simulink model "SRM_Project"  (R2025b)
settings: Solver=ode4  StartTime=0.0  StopTime=0.2  FixedStep=1e-5  RelTol=1e-3
InitFcn:
  | SRM_params
values from neighbouring files (symbols this model uses):
  B = 0.001    [SRM_params_template.m]
  delta_i = 0.1    [SRM_params_template.m]
  dLdth_vec = gradient(L_vec, theta_vec)    [SRM_params_template.m]
  Imax = 15    [SRM_params_template.m]
  J = 0.002    [SRM_params_template.m]
  Ki_w = 10    [SRM_params_template.m]
  Kp_w = 0.5    [SRM_params_template.m]
  L_vec = zeros(size(theta_vec))    [SRM_params_template.m]
  phase_offset = 2*pi/(Nph*Nr)    (= 0.523598775598)    [SRM_params_template.m]
  Rs = 1.0    (= 1)    [SRM_params_template.m]
  T_max = 5    [SRM_params_template.m]
  theta_off = deg2rad(38)    [SRM_params_template.m]
  theta_on = 0    [SRM_params_template.m]
  theta_ov = deg2rad(10)    [SRM_params_template.m]
  theta_vec = linspace(0, pi/2, 1000)    [SRM_params_template.m]
  TL = 1.5    [SRM_params_template.m]    (also in SRM_plots.m = out.TorqueData.signals(1).values(:, 2))
  tsf_type = 3    [SRM_params_template.m]
  Vdc = 300    [SRM_params_template.m]
libraries: slpidlib x1
settings Model: Creator=Dell  LastModifiedBy=Dell

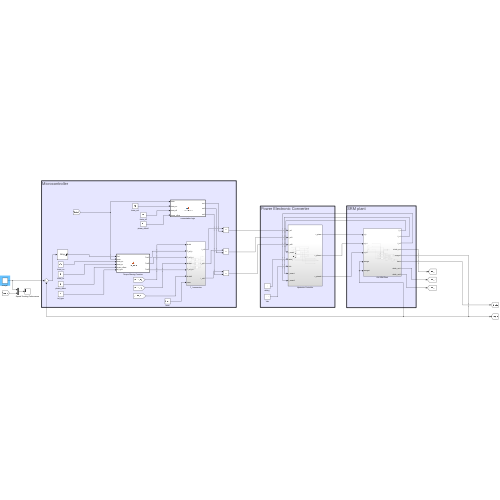
[thumbnail: Simulink's stored preview of the top-level diagram]
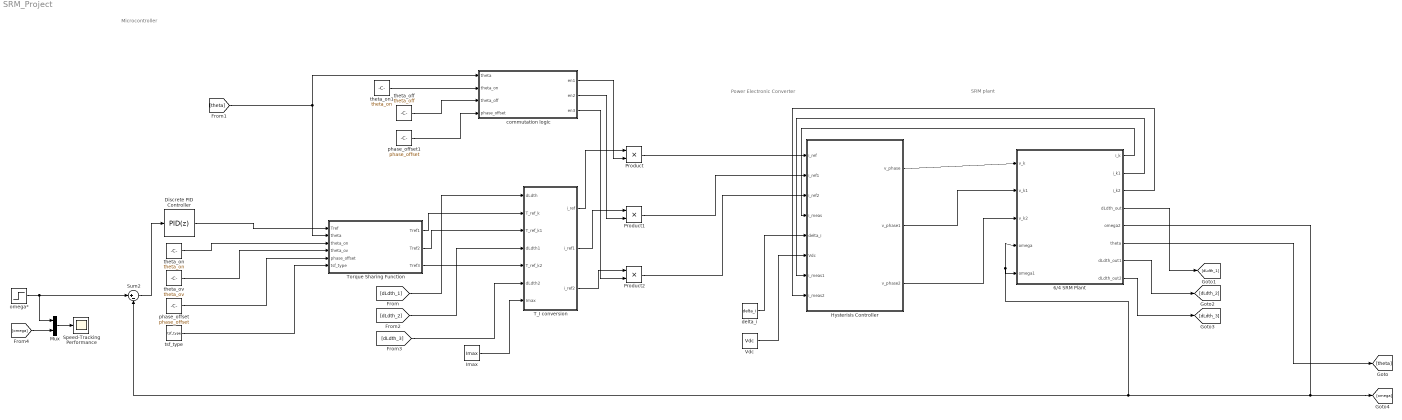
== system SRM_Project ==
  note: Power Electronic Converter
  note: Microcontroller
  note: SRM plant
  6/4 SRM Plant : Subsystem
  Discrete PID Controller : slpidlib/PID Controller  Controller=PID  Form=Parallel  TimeDomain=Discrete-time  UseExternalTs=off  SampleTime=-1  IntegratorMethod=Forward Euler  FilterMethod=Forward Euler  ControllerParametersSource=internal  P=Kp_w  I=Ki_w  UseKiTs=off  D=0  UseExternalDerivativeSource=off  N=100  UseFilter=on  TunerSelectOption=Transfer Function Based (PID Tuner App)  InitialConditionSource=internal  InitialConditionForIntegrator=0  InitialConditionForFilter=0  DifferentiatorICPrevScaledInput=0  ExternalReset=none  TrackingMode=off  Kt=1  LimitOutput=on  SatLimitsSource=internal  UpperSaturationLimit=T_max  LowerSaturationLimit=0  LinearizeAsGain=off  AntiWindupMode=none  Kb=1  LimitIntegrator=off  UpperIntegratorSaturationLimit=inf  LowerIntegratorSaturationLimit=-inf  POutMin=[]  POutMax=[]  IOutMin=[]  IOutMax=[]  DOutMin=[]  DOutMax=[]  NOutMin=[]  NOutMax=[]  SumOutMin=[]  SumOutMax=[]  SaturationOutMin=[]  SaturationOutMax=[]  PParamMin=[]  PParamMax=[]  IParamMin=[]  IParamMax=[]  DParamMin=[]  DParamMax=[]  NParamMin=[]  NParamMax=[]  KbParamMin=[]  KbParamMax=[]  KtParamMin=[]  KtParamMax=[]  KbOutMin=[]  KbOutMax=[]  KtOutMin=[]  KtOutMax=[]  IntegratorOutMin=[]  IntegratorOutMax=[]  FilterOutMin=[]  FilterOutMax=[]  SumI1OutMin=[]  SumI1OutMax=[]  SumI2OutMin=[]  SumI2OutMax=[]  SumI3OutMin=[]  SumI3OutMax=[]  SumI4OutMin=[]  SumI4OutMax=[]  SumDOutMin=[]  SumDOutMax=[]  DifferentiatorOutMin=[]  DifferentiatorOutMax=[]  FilterDiffOutCoefMin=[]  FilterDiffOutCoefMax=[]  ReciprocalOutMin=[]  ReciprocalOutMax=[]  SumDenOutMin=[]  SumDenOutMax=[]  SumNumOutMin=[]  SumNumOutMax=[]  DivideOutMin=[]  DivideOutMax=[]  UdiffTsProdOutMin=[]  UdiffTsProdOutMax=[]  NTsProdOutMin=[]  NTsProdOutMax=[]  UintegralTsProdOutMin=[]  UintegralTsProdOutMax=[]  UngainTsProdOutMin=[]  UngainTsProdOutMax=[]  ClampingZeroOutDataTypeStr=Inherit: Inherit via back propagation  ClampingZeroOutMin=[]  ClampingZeroOutMax=[]  FilterDenConstantOutDataTypeStr=Inherit: Inherit via back propagation  FilterDenConstantOutMin=[]  FilterDenConstantOutMax=[]  PCopyOutDataTypeStr=Inherit: Inherit via back propagation  PCopyOutMin=[]  PCopyOutMax=[]  NCopyOutDataTypeStr=Inherit: Inherit via back propagation  NCopyOutMin=[]  NCopyOutMax=[]  IntegratorContinuousStateAttributes=''  IntegratorStateMustResolveToSignalObject=off  IntegratorRTWStateStorageClass=Auto  FilterContinuousStateAttributes=''  FilterStateMustResolveToSignalObject=off  FilterRTWStateStorageClass=Auto  ParallelPVariant=InternalParameters  IdealPVariant=Disabled  IVariant=InternalParameters  DVariant=InternalParameters  IntegratorVariant=Discrete  SatVariant=Enabled  AWVariant=Passthrough  PCopyVariant=Disabled  TRVariant=Disabled  FdbkBlocksVariant=Forward  IdealPFdbkVariant=Disabled  SatFdbkVariant=Disabled  DerivativeFilterVariant=ForwardEulerFilter  NVariant=InternalParameters  NCopyVariant=Disabled  FilterICVariant=InternalICsFilter  IntegratorICVariant=InternalICs  ExternalResetVariant=Disabled  TRSumVariant=Passthrough  SumFdbkVariant=Disabled  SumVariant=Sum_PID  TsampFilterVariant=InternalTs  TsampNgainVariant=Passthrough  TsampIntegralVariant=Disabled_SignalSpec  ExternalSaturationOutDataTypeStr=Inherit: Same as second input  DerivativeSourceVariant=ErrorSignal  PreIntVariant=InternalPreInt
      settings: LibrarySourceBlock=simulink/Discrete/Discrete PID Controller
  Hysterisis Controller : Subsystem
  Imax : Constant  Value=Imax
  Mux : Mux  Inputs=2
  Product : Product
  Product1 : Product
  Product2 : Product
  Speed-Tracking Performance : Scope
      settings: Title=Speed Tracking Performance  ActiveDisplayYMinimum=-84.626335167126086  ActiveDisplayYMaximum=313.00000660773765  YLabel=Omega  DataLoggingVariableName=SpeedData
  Sum2 : Sum  Inputs=|+-
  T_I conversion : Subsystem
  Torque Sharing Function : MATLAB Function  TreatAsAtomicUnit=on
  Vdc : Constant  Value=Vdc
  commutation logic : MATLAB Function  TreatAsAtomicUnit=on
  delta_i : Constant  Value=delta_i
  omega* : Step  Time=0  After=100  SampleTime=0
  phase_offset : Constant  Value=phase_offset
  phase_offset1 : Constant  Value=phase_offset
  theta_off : Constant  Value=theta_off
  theta_on : Constant  Value=theta_on
  theta_on1 : Constant  Value=theta_on
  theta_ov : Constant  Value=theta_ov
  tsf_type : Constant  Value=tsf_type
  wires:
  omega*/1 -> Mux/1, Sum2/1
  Sum2/1 -> Discrete PID Controller/1
  Discrete PID Controller/1 -> Torque Sharing Function/1(Tref)
  commutation logic/1(en1) -> Product/2
  commutation logic/2(en2) -> Product1/2
  commutation logic/3(en3) -> Product2/2
  [theta] -> Torque Sharing Function/2(theta), commutation logic/1(theta)
  theta_on/1 -> Torque Sharing Function/3(theta_on)
  theta_ov/1 -> Torque Sharing Function/4(theta_ov)
  theta_on1/1 -> commutation logic/2(theta_on)
  phase_offset/1 -> Torque Sharing Function/5(phase_offset)
  phase_offset1/1 -> commutation logic/4(phase_offset)
  tsf_type/1 -> Torque Sharing Function/6(tsf_type)
  theta_off/1 -> commutation logic/3(theta_off)
  [omega] -> Mux/2
  Mux/1 -> Speed-Tracking Performance/1
  Product/1 -> Hysterisis Controller/1(i_ref)
  Product1/1 -> Hysterisis Controller/2(i_ref1)
  Product2/1 -> Hysterisis Controller/3(i_ref2)
  delta_i/1 -> Hysterisis Controller/5(delta_i)
  Vdc/1 -> Hysterisis Controller/6(Vdc)
  6/4 SRM Plant/5(omega2) -> [omega], 6/4 SRM Plant/4(omega), 6/4 SRM Plant/5(omega1), Sum2/2
  Hysterisis Controller/1(v_phase) -> 6/4 SRM Plant/1(v_k)
  Hysterisis Controller/2(v_phase1) -> 6/4 SRM Plant/2(v_k1)
  Hysterisis Controller/3(v_phase2) -> 6/4 SRM Plant/3(v_k2)
  6/4 SRM Plant/1(i_k) -> Hysterisis Controller/4(i_meas)
  6/4 SRM Plant/2(i_k1) -> Hysterisis Controller/7(i_meas1)
  6/4 SRM Plant/3(i_k2) -> Hysterisis Controller/8(i_meas2)
  6/4 SRM Plant/4(dLdth_out) -> [dLdth_1]
  6/4 SRM Plant/6(theta) -> [theta]
  6/4 SRM Plant/7(dLdth_out1) -> [dLdth_2]
  6/4 SRM Plant/8(dLdth_out2) -> [dLdth_3]
  [dLdth_1] -> T_I conversion/1(dLdth)
  Torque Sharing Function/1(Tref1) -> T_I conversion/2(T_ref_k)
  Torque Sharing Function/2(Tref2) -> T_I conversion/3(T_ref_k1)
  [dLdth_2] -> T_I conversion/4(dLdth1)
  Torque Sharing Function/3(Tref3) -> T_I conversion/5(T_ref_k2)
  [dLdth_3] -> T_I conversion/6(dLdth2)
  Imax/1 -> T_I conversion/7(Imax)
  T_I conversion/1(i_ref) -> Product/1
  T_I conversion/2(i_ref1) -> Product1/1
  T_I conversion/3(i_ref2) -> Product2/1

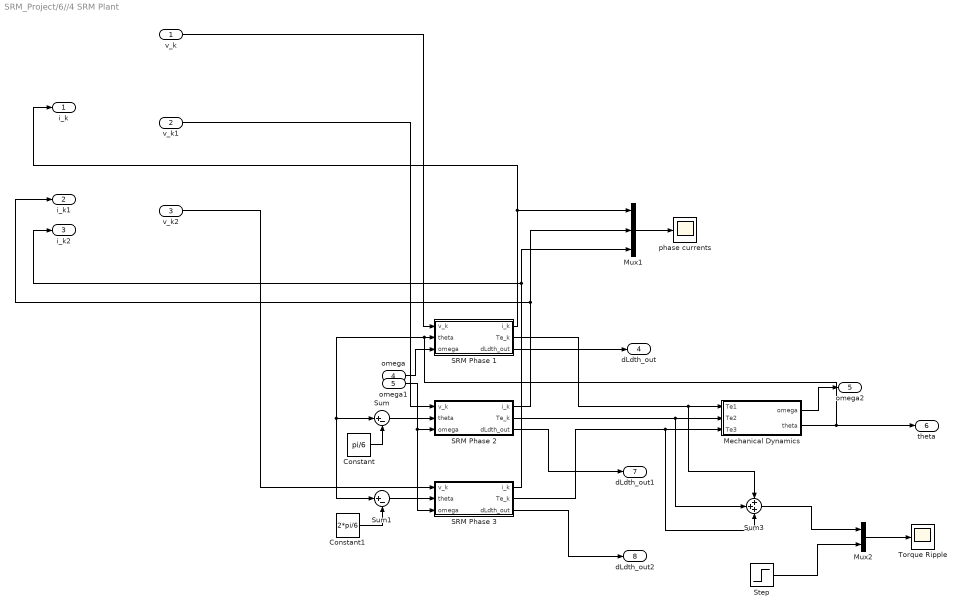
== system SRM_Project/6//4 SRM Plant ==
  v_k : Inport
  v_k1 : Inport  Port=2
  v_k2 : Inport  Port=3
  omega : Inport  Port=4
  omega1 : Inport  Port=5
  Constant : Constant  Value=pi/6
  Constant1 : Constant  Value=2*pi/6
  Mechanical Dynamics : Subsystem
  Mux1 : Mux  Inputs=3
  Mux2 : Mux  Inputs=2
  SRM Phase 1 : Subsystem
  SRM Phase 2 : Subsystem
  SRM Phase 3 : Subsystem
  Step : Step  Time=0.1  After=TL  SampleTime=0
  Sum : Sum  Inputs=|+-
  Sum1 : Sum  Inputs=|+-
  Sum3 : Sum  Inputs=+++
  Torque Ripple : Scope
      settings: ActiveDisplayYMinimum=-0.28454912524967474  ActiveDisplayYMaximum=2.8390389361123889  DataLoggingVariableName=TorqueData
  phase currents : Scope
      settings: ActiveDisplayYMinimum=-0.63560077718964481  ActiveDisplayYMaximum=5.7204069947068081  DataLoggingVariableName=CurrentData
  i_k : Outport
  i_k1 : Outport  Port=2
  i_k2 : Outport  Port=3
  dLdth_out : Outport  Port=4
  omega2 : Outport  Port=5
  theta : Outport  Port=6
  dLdth_out1 : Outport  Port=7
  dLdth_out2 : Outport  Port=8
  wires:
  Mechanical Dynamics/2(theta) -> theta/1, Sum/1, Sum1/1, SRM Phase 1/2(theta)
  Mux1/1 -> phase currents/1
  Sum1/1 -> SRM Phase 3/2(theta)
  SRM Phase 1/2(Te_k) -> Sum3/1, Mechanical Dynamics/1(Te1)
  v_k2/1 -> SRM Phase 3/1(v_k)
  SRM Phase 2/2(Te_k) -> Sum3/2, Mechanical Dynamics/2(Te2)
  Mechanical Dynamics/1(omega) -> omega2/1
  Sum/1 -> SRM Phase 2/2(theta)
  Constant1/1 -> Sum1/2
  Sum3/1 -> Mux2/1
  omega1/1 -> SRM Phase 3/3(omega), SRM Phase 2/3(omega)
  SRM Phase 3/1(i_k) -> i_k2/1, Mux1/3
  Constant/1 -> Sum/2
  SRM Phase 3/2(Te_k) -> Sum3/3, Mechanical Dynamics/3(Te3)
  Mux2/1 -> Torque Ripple/1
  SRM Phase 2/1(i_k) -> i_k1/1, Mux1/2
  SRM Phase 3/3(dLdth_out) -> dLdth_out2/1
  v_k1/1 -> SRM Phase 2/1(v_k)
  Step/1 -> Mux2/2
  SRM Phase 1/1(i_k) -> i_k/1, Mux1/1
  SRM Phase 1/3(dLdth_out) -> dLdth_out/1
  SRM Phase 2/3(dLdth_out) -> dLdth_out1/1
  omega/1 -> SRM Phase 1/3(omega)
  v_k/1 -> SRM Phase 1/1(v_k)

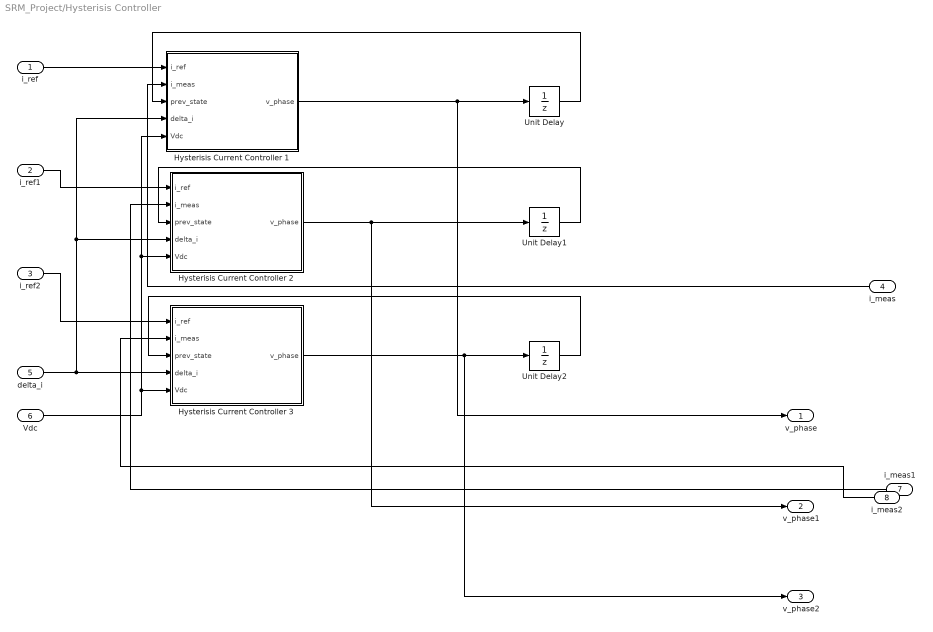
== system SRM_Project/Hysterisis Controller ==
  i_ref : Inport
  i_ref1 : Inport  Port=2
  i_ref2 : Inport  Port=3
  i_meas : Inport  Port=4
  delta_i : Inport  Port=5
  Vdc : Inport  Port=6
  i_meas1 : Inport  Port=7
  i_meas2 : Inport  Port=8
  Hysterisis Current Controller 1 : MATLAB Function  TreatAsAtomicUnit=on
  Hysterisis Current Controller 2 : MATLAB Function  TreatAsAtomicUnit=on
  Hysterisis Current Controller 3 : MATLAB Function  TreatAsAtomicUnit=on
  Unit Delay : UnitDelay  SampleTime=-1  HasFrameUpgradeWarning=on
  Unit Delay1 : UnitDelay  SampleTime=-1  HasFrameUpgradeWarning=on
  Unit Delay2 : UnitDelay  SampleTime=-1  HasFrameUpgradeWarning=on
  v_phase : Outport
  v_phase1 : Outport  Port=2
  v_phase2 : Outport  Port=3
  wires:
  Vdc/1 -> Hysterisis Current Controller 1/5(Vdc), Hysterisis Current Controller 2/5(Vdc), Hysterisis Current Controller 3/5(Vdc)
  Unit Delay1/1 -> Hysterisis Current Controller 2/3(prev_state)
  Hysterisis Current Controller 2/1(v_phase) -> v_phase1/1, Unit Delay1/1
  delta_i/1 -> Hysterisis Current Controller 3/4(delta_i), Hysterisis Current Controller 1/4(delta_i), Hysterisis Current Controller 2/4(delta_i)
  Hysterisis Current Controller 1/1(v_phase) -> v_phase/1, Unit Delay/1
  Unit Delay/1 -> Hysterisis Current Controller 1/3(prev_state)
  Hysterisis Current Controller 3/1(v_phase) -> v_phase2/1, Unit Delay2/1
  i_meas1/1 -> Hysterisis Current Controller 2/2(i_meas)
  i_ref1/1 -> Hysterisis Current Controller 2/1(i_ref)
  Unit Delay2/1 -> Hysterisis Current Controller 3/3(prev_state)
  i_ref/1 -> Hysterisis Current Controller 1/1(i_ref)
  i_ref2/1 -> Hysterisis Current Controller 3/1(i_ref)
  i_meas2/1 -> Hysterisis Current Controller 3/2(i_meas)
  i_meas/1 -> Hysterisis Current Controller 1/2(i_meas)

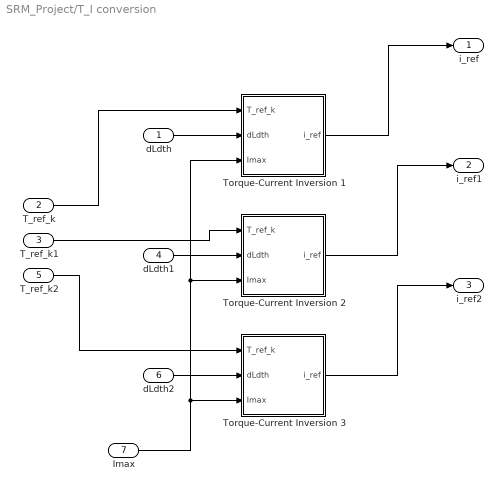
== system SRM_Project/T_I conversion ==
  dLdth : Inport
  T_ref_k : Inport  Port=2
  T_ref_k1 : Inport  Port=3
  dLdth1 : Inport  Port=4
  T_ref_k2 : Inport  Port=5
  dLdth2 : Inport  Port=6
  Imax : Inport  Port=7
  Torque-Current Inversion 1 : MATLAB Function  TreatAsAtomicUnit=on
  Torque-Current Inversion 2 : MATLAB Function  TreatAsAtomicUnit=on
  Torque-Current Inversion 3 : MATLAB Function  TreatAsAtomicUnit=on
  i_ref : Outport
  i_ref1 : Outport  Port=2
  i_ref2 : Outport  Port=3
  wires:
  dLdth1/1 -> Torque-Current Inversion 2/2(dLdth)
  dLdth/1 -> Torque-Current Inversion 1/2(dLdth)
  Imax/1 -> Torque-Current Inversion 1/3(Imax), Torque-Current Inversion 2/3(Imax), Torque-Current Inversion 3/3(Imax)
  T_ref_k1/1 -> Torque-Current Inversion 2/1(T_ref_k)
  T_ref_k/1 -> Torque-Current Inversion 1/1(T_ref_k)
  Torque-Current Inversion 2/1(i_ref) -> i_ref1/1
  Torque-Current Inversion 3/1(i_ref) -> i_ref2/1
  Torque-Current Inversion 1/1(i_ref) -> i_ref/1
  T_ref_k2/1 -> Torque-Current Inversion 3/1(T_ref_k)
  dLdth2/1 -> Torque-Current Inversion 3/2(dLdth)

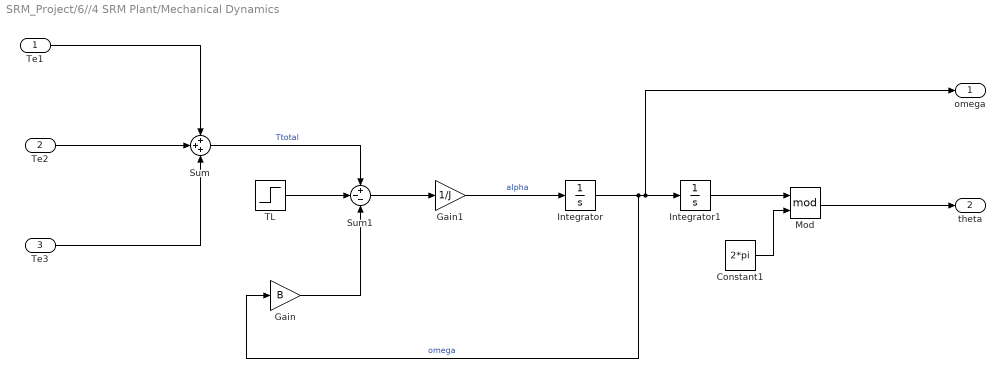
== system SRM_Project/6//4 SRM Plant/Mechanical Dynamics ==
  Te1 : Inport
  Te2 : Inport  Port=2
  Te3 : Inport  Port=3
  Constant1 : Constant  Value=2*pi
  Gain : Gain  Gain=B
  Gain1 : Gain  Gain=1/J
  Integrator : Integrator
  Integrator1 : Integrator
  Mod : Math  Operator=mod
  Sum : Sum  Inputs=+++
  Sum1 : Sum  Inputs=+--
  TL : Step  Time=0.1  After=TL  SampleTime=0
  omega : Outport
  theta : Outport  Port=2
  wires:
  Te2/1 -> Sum/2
  Te1/1 -> Sum/1
  Te3/1 -> Sum/3
  Sum/1 -> Sum1/1  "Ttotal"
  TL/1 -> Sum1/2
  Gain/1 -> Sum1/3
  Sum1/1 -> Gain1/1
  Gain1/1 -> Integrator/1  "alpha"
  Integrator/1 -> Integrator1/1, omega/1, Gain/1  "omega"
  Integrator1/1 -> Mod/1
  Constant1/1 -> Mod/2
  Mod/1 -> theta/1

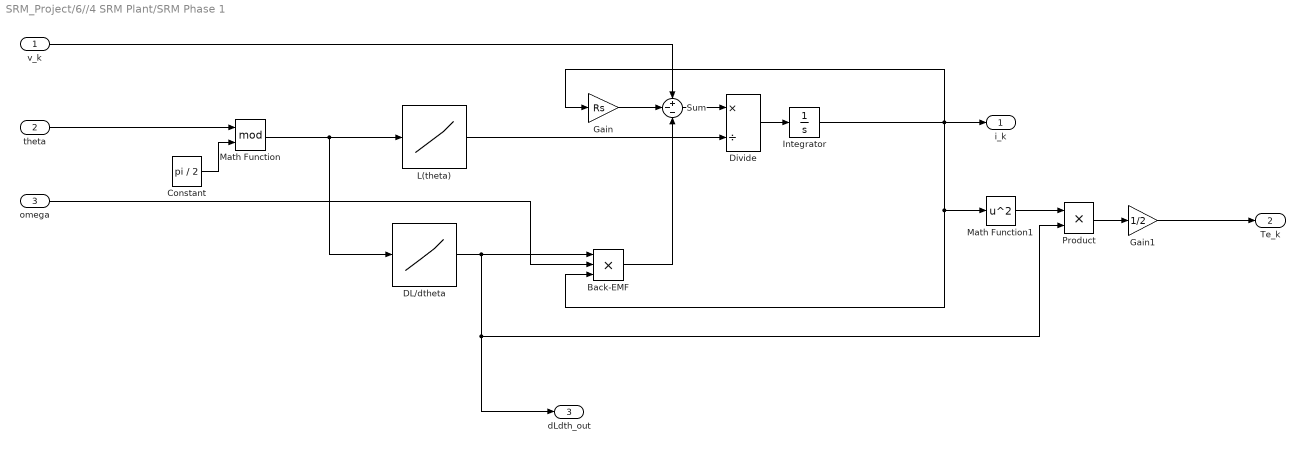
== system SRM_Project/6//4 SRM Plant/SRM Phase 1 ==
  v_k : Inport
  theta : Inport  Port=2
  omega : Inport  Port=3
  Back-EMF : Product  Inputs=3
  Constant : Constant  Value=pi / 2
  DL/dtheta : Lookup_n-D  NumberOfTableDimensions=1  BreakpointsForDimension1=theta_vec  Table=dLdth_vec  InternalRulePriority=Speed  RndMeth=Simplest
  Divide : Product  Inputs=*/
  Gain : Gain  Gain=Rs
  Gain1 : Gain  Gain=1/2
  Integrator : Integrator  LimitOutput=on  LowerSaturationLimit=0
  L(theta) : Lookup_n-D  NumberOfTableDimensions=1  BreakpointsForDimension1=theta_vec  Table=L_vec  InternalRulePriority=Speed  RndMeth=Simplest
  Math Function : Math  Operator=mod
  Math Function1 : Math  Operator=square
  Product : Product
  Sum : Sum  Inputs=+--
  i_k : Outport
  Te_k : Outport  Port=2
  dLdth_out : Outport  Port=3
  wires:
  theta/1 -> Math Function/1
  Constant/1 -> Math Function/2
  Math Function/1 -> DL/dtheta/1, L(theta)/1
  omega/1 -> Back-EMF/2
  DL/dtheta/1 -> dLdth_out/1, Product/2, Back-EMF/1
  v_k/1 -> Sum/1
  Gain/1 -> Sum/2
  Back-EMF/1 -> Sum/3
  Sum/1 -> Divide/1
  L(theta)/1 -> Divide/2
  Divide/1 -> Integrator/1
  Integrator/1 -> Math Function1/1, Back-EMF/3, i_k/1, Gain/1
  Math Function1/1 -> Product/1
  Product/1 -> Gain1/1
  Gain1/1 -> Te_k/1

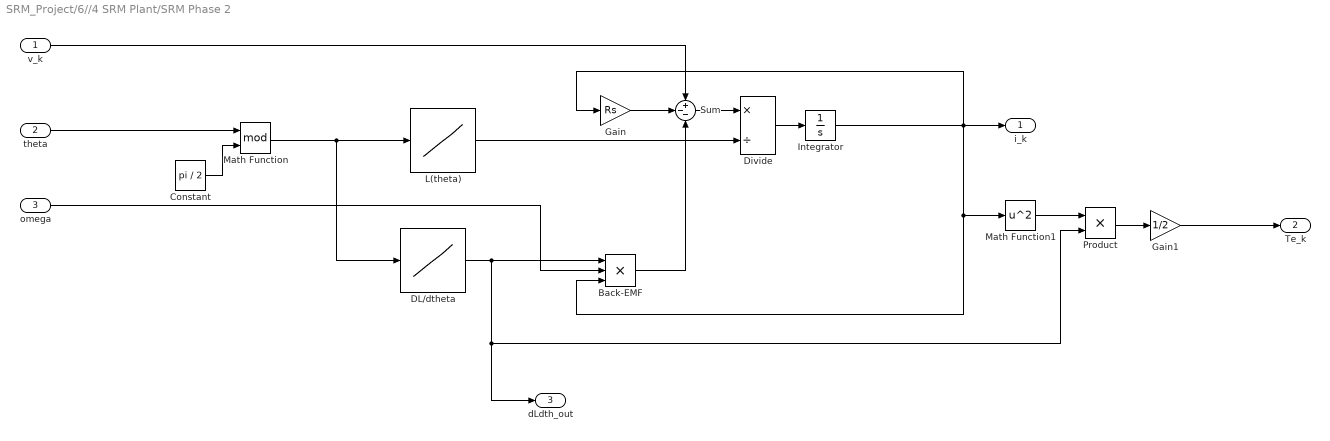
== system SRM_Project/6//4 SRM Plant/SRM Phase 2 ==
  v_k : Inport
  theta : Inport  Port=2
  omega : Inport  Port=3
  Back-EMF : Product  Inputs=3
  Constant : Constant  Value=pi / 2
  DL/dtheta : Lookup_n-D  NumberOfTableDimensions=1  BreakpointsForDimension1=theta_vec  Table=dLdth_vec  InternalRulePriority=Speed  RndMeth=Simplest
  Divide : Product  Inputs=*/
  Gain : Gain  Gain=Rs
  Gain1 : Gain  Gain=1/2
  Integrator : Integrator  LimitOutput=on  LowerSaturationLimit=0
  L(theta) : Lookup_n-D  NumberOfTableDimensions=1  BreakpointsForDimension1=theta_vec  Table=L_vec  InternalRulePriority=Speed  RndMeth=Simplest
  Math Function : Math  Operator=mod
  Math Function1 : Math  Operator=square
  Product : Product
  Sum : Sum  Inputs=+--
  i_k : Outport
  Te_k : Outport  Port=2
  dLdth_out : Outport  Port=3
  wires:
  theta/1 -> Math Function/1
  Constant/1 -> Math Function/2
  Math Function/1 -> DL/dtheta/1, L(theta)/1
  omega/1 -> Back-EMF/2
  DL/dtheta/1 -> dLdth_out/1, Product/2, Back-EMF/1
  v_k/1 -> Sum/1
  Gain/1 -> Sum/2
  Back-EMF/1 -> Sum/3
  Sum/1 -> Divide/1
  L(theta)/1 -> Divide/2
  Divide/1 -> Integrator/1
  Integrator/1 -> Math Function1/1, Back-EMF/3, i_k/1, Gain/1
  Math Function1/1 -> Product/1
  Product/1 -> Gain1/1
  Gain1/1 -> Te_k/1

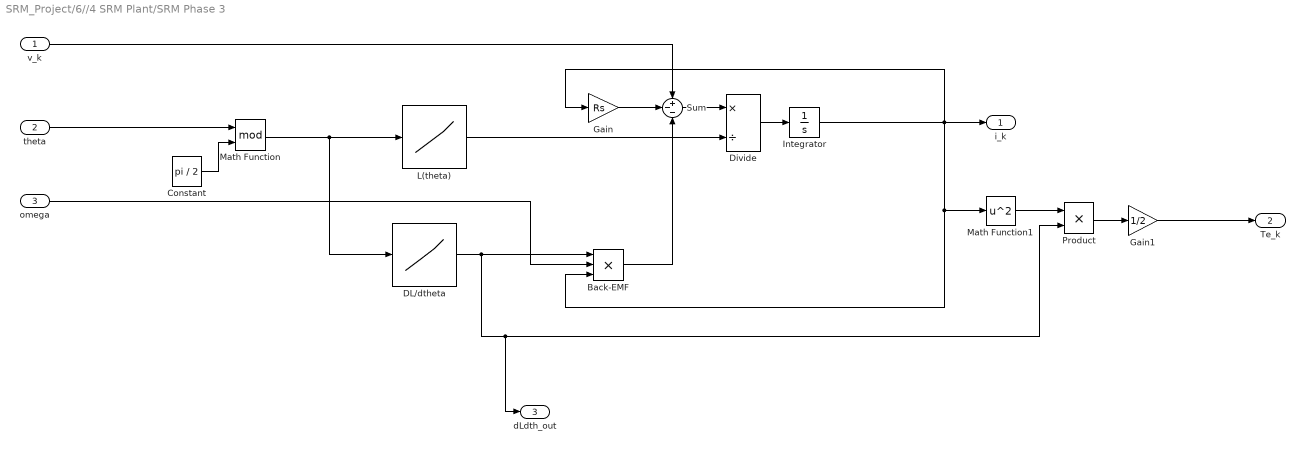
== system SRM_Project/6//4 SRM Plant/SRM Phase 3 ==
  v_k : Inport
  theta : Inport  Port=2
  omega : Inport  Port=3
  Back-EMF : Product  Inputs=3
  Constant : Constant  Value=pi / 2
  DL/dtheta : Lookup_n-D  NumberOfTableDimensions=1  BreakpointsForDimension1=theta_vec  Table=dLdth_vec  InternalRulePriority=Speed  RndMeth=Simplest
  Divide : Product  Inputs=*/
  Gain : Gain  Gain=Rs
  Gain1 : Gain  Gain=1/2
  Integrator : Integrator  LimitOutput=on  LowerSaturationLimit=0
  L(theta) : Lookup_n-D  NumberOfTableDimensions=1  BreakpointsForDimension1=theta_vec  Table=L_vec  InternalRulePriority=Speed  RndMeth=Simplest
  Math Function : Math  Operator=mod
  Math Function1 : Math  Operator=square
  Product : Product
  Sum : Sum  Inputs=+--
  i_k : Outport
  Te_k : Outport  Port=2
  dLdth_out : Outport  Port=3
  wires:
  theta/1 -> Math Function/1
  Constant/1 -> Math Function/2
  Math Function/1 -> DL/dtheta/1, L(theta)/1
  omega/1 -> Back-EMF/2
  DL/dtheta/1 -> dLdth_out/1, Product/2, Back-EMF/1
  v_k/1 -> Sum/1
  Gain/1 -> Sum/2
  Back-EMF/1 -> Sum/3
  Sum/1 -> Divide/1
  L(theta)/1 -> Divide/2
  Divide/1 -> Integrator/1
  Integrator/1 -> Math Function1/1, Back-EMF/3, i_k/1, Gain/1
  Math Function1/1 -> Product/1
  Product/1 -> Gain1/1
  Gain1/1 -> Te_k/1

== matlab function SRM_Project/Torque Sharing Function ==
  data: Tref input; Tref1 output; theta input; theta_on input; theta_ov input; phase_offset input; tsf_type input; Tref2 output; Tref3 output
function [Tref1, Tref2, Tref3] = TSF_Block(Tref, theta, theta_on, theta_ov, phase_offset, tsf_type)
    pp = pi/2;
    refs = zeros(1,3);
    
    for k = 1:3
        th = mod(theta - (k-1)*phase_offset, pp);
        
        % Rising portion (incoming phase)
        if th >= theta_on && th <= (theta_on + theta_ov)
            x = (th - theta_on)/theta_ov;
            fr = TSF_rising(x, tsf_type);
            refs(k) = fr * Tref;
            
        % Full conduction
        elseif th > (theta_on + theta_ov) && th <= (theta_on + pp/2)
            refs(k) = Tref;
            
        % Falling portion (outgoing phase)
        elseif th > (theta_on + pp/2) && th <= (theta_on + pp/2 + theta_ov)
            x = (th - (theta_on + pp/2))/theta_ov;
            refs(k) = (1 - TSF_rising(x, tsf_type)) * Tref;
            
        else
            refs(k) = 0;
        end
    end
    
    Tref1 = refs(1); Tref2 = refs(2); Tref3 = refs(3);
end

function fr = TSF_rising(x, type)
    switch type
        case 1, fr = x;                           % Linear
        case 2, fr = 0.5*(1 - cos(pi*x));         % Sinusoidal
        case 3, fr = 3*x^2 - 2*x^3;               % Cubic
        case 4, fr = 1 - exp(-3*x);               % Exponential
        otherwise, fr = x;
    end
    fr = min(max(fr, 0), 1); % Bound between 0 and 1
end

== matlab function SRM_Project/commutation logic ==
  data: theta input; en1 output; theta_on input; theta_off input; phase_offset input; en2 output; en3 output
function [en1, en2, en3] = commutation(theta, theta_on, theta_off, phase_offset)
    % Wrap angle to one pole pitch
    pp = pi/2; 
    th1 = mod(theta, pp);
    th2 = mod(theta - phase_offset, pp);
    th3 = mod(theta - 2*phase_offset, pp);
    
    % Generate boolean enable signals
    en1 = double(th1 >= theta_on && th1 <= theta_off);
    en2 = double(th2 >= theta_on && th2 <= theta_off);
    en3 = double(th3 >= theta_on && th3 <= theta_off);
end

== matlab function SRM_Project/T_I conversion/Torque-Current Inversion 1 ==
  data: T_ref_k input; i_ref output; dLdth input; Imax input
function i_ref = T_to_I(T_ref_k, dLdth, Imax)
    % 1. Force torque reference to be zero or positive
    T_clean = max(0, T_ref_k);
    
    % 2. Prevent division by zero and get the absolute slope
    slope = max(abs(dLdth), 1e-6);
    
    % 3. The Bulletproof Line: abs() inside the sqrt guarantees 
    % to the Simulink compiler that the output is strictly Real.
    i_ref = sqrt(abs(2 * T_clean / slope));
    
    % 4. Apply hardware limits
    i_ref = min(i_ref, Imax);
end

== matlab function SRM_Project/Hysterisis Controller/Hysterisis Current Controller 1 ==
  data: i_ref input; v_phase output; i_meas input; prev_state input; delta_i input; Vdc input
function v_phase = hysteresis_ctrl(i_ref, i_meas, prev_state, delta_i, Vdc)
    % prev_state is fed back via a Unit Delay block
    if i_meas < (i_ref - delta_i/2)
        v_phase = Vdc;        % Magnetize phase
    elseif i_meas > (i_ref + delta_i/2)
        v_phase = -Vdc;       % Demagnetize phase (return energy)
    else
        v_phase = prev_state; % Freewheel / hold state
    end
end

== matlab function SRM_Project/T_I conversion/Torque-Current Inversion 2 ==
  data: T_ref_k input; i_ref output; dLdth input; Imax input
function i_ref = T_to_I(T_ref_k, dLdth, Imax)
    % 1. Force torque reference to be zero or positive
    T_clean = max(0, T_ref_k);
    
    % 2. Prevent division by zero and get the absolute slope
    slope = max(abs(dLdth), 1e-6);
    
    % 3. The Bulletproof Line: abs() inside the sqrt guarantees 
    % to the Simulink compiler that the output is strictly Real.
    i_ref = sqrt(abs(2 * T_clean / slope));
    
    % 4. Apply hardware limits
    i_ref = min(i_ref, Imax);
end

== matlab function SRM_Project/T_I conversion/Torque-Current Inversion 3 ==
  data: T_ref_k input; i_ref output; dLdth input; Imax input
function i_ref = T_to_I(T_ref_k, dLdth, Imax)
    % 1. Force torque reference to be zero or positive
    T_clean = max(0, T_ref_k);
    
    % 2. Prevent division by zero and get the absolute slope
    slope = max(abs(dLdth), 1e-6);
    
    % 3. The Bulletproof Line: abs() inside the sqrt guarantees 
    % to the Simulink compiler that the output is strictly Real.
    i_ref = sqrt(abs(2 * T_clean / slope));
    
    % 4. Apply hardware limits
    i_ref = min(i_ref, Imax);
end

== matlab function SRM_Project/Hysterisis Controller/Hysterisis Current Controller 2 ==
  data: i_ref input; v_phase output; i_meas input; prev_state input; delta_i input; Vdc input
function v_phase = hysteresis_ctrl(i_ref, i_meas, prev_state, delta_i, Vdc)
    % prev_state is fed back via a Unit Delay block
    if i_meas < (i_ref - delta_i/2)
        v_phase = Vdc;        % Magnetize phase
    elseif i_meas > (i_ref + delta_i/2)
        v_phase = -Vdc;       % Demagnetize phase (return energy)
    else
        v_phase = prev_state; % Freewheel / hold state
    end
end

== matlab function SRM_Project/Hysterisis Controller/Hysterisis Current Controller 3 ==
  data: i_ref input; v_phase output; i_meas input; prev_state input; delta_i input; Vdc input
function v_phase = hysteresis_ctrl(i_ref, i_meas, prev_state, delta_i, Vdc)
    % prev_state is fed back via a Unit Delay block
    if i_meas < (i_ref - delta_i/2)
        v_phase = Vdc;        % Magnetize phase
    elseif i_meas > (i_ref + delta_i/2)
        v_phase = -Vdc;       % Demagnetize phase (return energy)
    else
        v_phase = prev_state; % Freewheel / hold state
    end
end
